simulink model "exp12"  (R2025b)
settings: Solver=VariableStepAuto  StartTime=0.0  StopTime=10.0  RelTol=1e-3
settings Model: Creator=SUBHASH  LastModifiedBy=SUBHASH

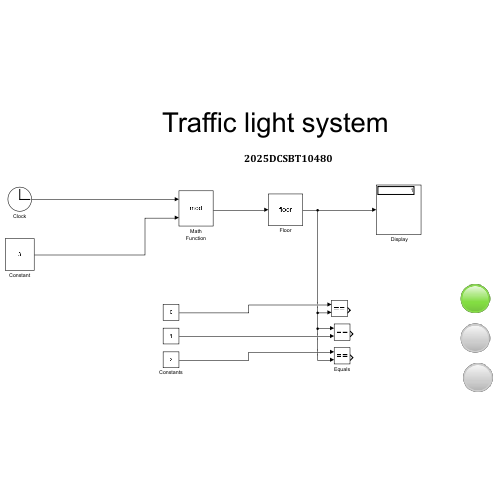
[thumbnail: Simulink's stored preview of the top-level diagram]
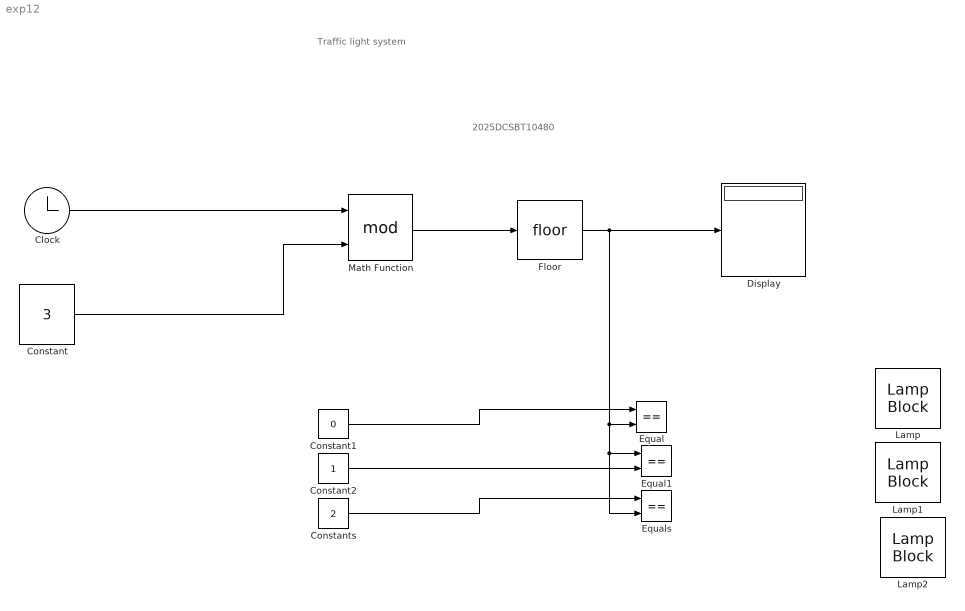
== system exp12 ==
  note: Traffic light system
  note: 2025DCSBT10480
  " Display" : Display
  Clock : Clock
  Constant : Constant  Value=3
  Constant1 : Constant  Value=0
  Constant2 : Constant
  Constants : Constant  Value=2
  Equal : RelationalOperator  Operator===  OutDataTypeStr=boolean  RndMeth=Simplest  InputSameDT=off
  Equal1 : RelationalOperator  Operator===  OutDataTypeStr=boolean  RndMeth=Simplest  InputSameDT=off
  Equals : RelationalOperator  Operator===  OutDataTypeStr=boolean  RndMeth=Simplest  InputSameDT=off
  Floor : Rounding
  Lamp : LampBlock  LabelPosition=Hide  DefaultColor=[192.0, 192.0, 192.0]
  Lamp1 : LampBlock  LabelPosition=Hide  DefaultColor=[192.0, 192.0, 192.0]
  Lamp2 : LampBlock  LabelPosition=Hide  DefaultColor=[192.0, 192.0, 192.0]
  Math Function : Math  Operator=mod
  wires:
  Clock/1 -> Math Function/1
  Constant/1 -> Math Function/2
  Math Function/1 -> Floor/1
  Constant2/1 -> Equal1/2
  Floor/1 -> " Display"/1, Equal/2, Equal1/1, Equals/2
  Constants/1 -> Equals/1
  Constant1/1 -> Equal/1
